simulink model "Add_model"  (R2023b)
settings: Solver=FixedStepAuto  StartTime=0.0  StopTime=10.0  FixedStep=1  RelTol=1e-3
settings Model: Creator=40523  LastModifiedBy=40523
settings OptimizationCC: DefaultParameterBehavior=Inlined  EnhancedBackFolding=on  PassReuseOutputArgsAs=Individual arguments  ZeroExternalMemoryAtStartup=off  ZeroInternalMemoryAtStartup=off  OptimizeBlockOrder=speed  DifferentSizesBufferReuse=on  OptimizationCustomize=off  EfficientTunableParamExpr=on
settings DebuggingCC: ParameterTunabilityLossMsg=error
settings SFSimCC: MATLABDynamicMemAlloc=off
settings RTWCC: Description=Embedded Coder  SystemTargetFile=ert.tlc  TemplateMakefile=ert_default_tmf
settings CodeAppCC: ForceParamTrailComments=on  IgnoreCustomStorageClasses=off  OperatorAnnotations=on  SimulinkDataObjDesc=on  SFDataObjDesc=on  InsertBlockDesc=on
settings ERTTargetCC: TargetLangStandard=C99 (ISO)  GenerateSampleERTMain=on  InlinedParameterPlacement=NonHierarchical  ERTCustomFileTemplate=example_file_process.tlc

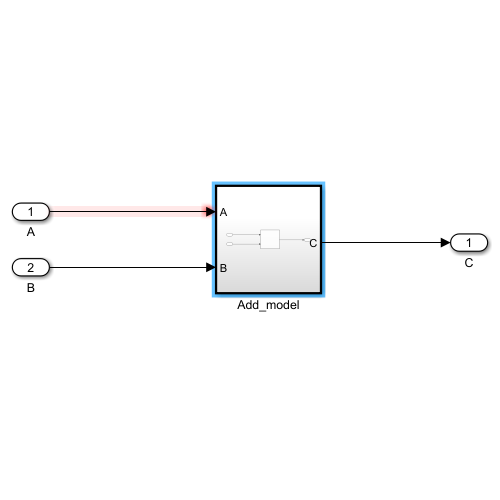
[thumbnail: Simulink's stored preview of the top-level diagram]
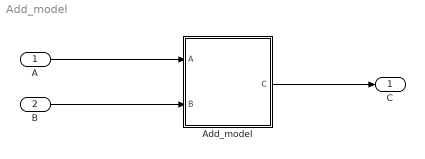
== system Add_model ==
  A : Inport  OutDataTypeStr=double
  B : Inport  Port=2  OutDataTypeStr=double
  Add_model : Subsystem  TreatAsAtomicUnit=on
  C : Outport  OutDataTypeStr=double
  wires:
  A/1 -> Add_model/1(A)
  B/1 -> Add_model/2(B)
  Add_model/1(C) -> C/1

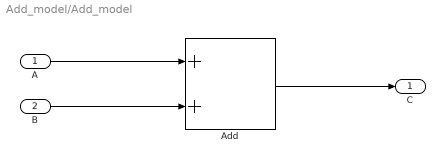
== system Add_model/Add_model ==
  A : Inport  OutDataTypeStr=double
  B : Inport  Port=2  OutDataTypeStr=double
  Add : Sum  OutDataTypeStr=double
  C : Outport  OutDataTypeStr=double
  wires:
  B/1 -> Add/2
  A/1 -> Add/1
  Add/1 -> C/1
